simulink model "simulacaoESC2DOF_SIAC"  (R2015a)
settings: Solver=ode4  StartTime=0.0  StopTime=120  FixedStep=0.001  RelTol=1e-3
values from neighbouring files (symbols this model uses):
  ampSenoide = 20    [simuOrientacaoESC.m]
  ampSenoide2 = 20    [simuOrientacaoESC.m]
  freqSenoide = 4*2*pi    (= 25.1327412287)    [simuOrientacaoESC.m]
  K = 1    [simuOrientacaoESC.m]
  Kp = 10    [simuOrientacaoESC.m]
undefined symbols (not defined in the file or in its folder): xL0
libraries: simulink_extras x5
settings Model: Creator=Jean  LastModifiedBy=Jean

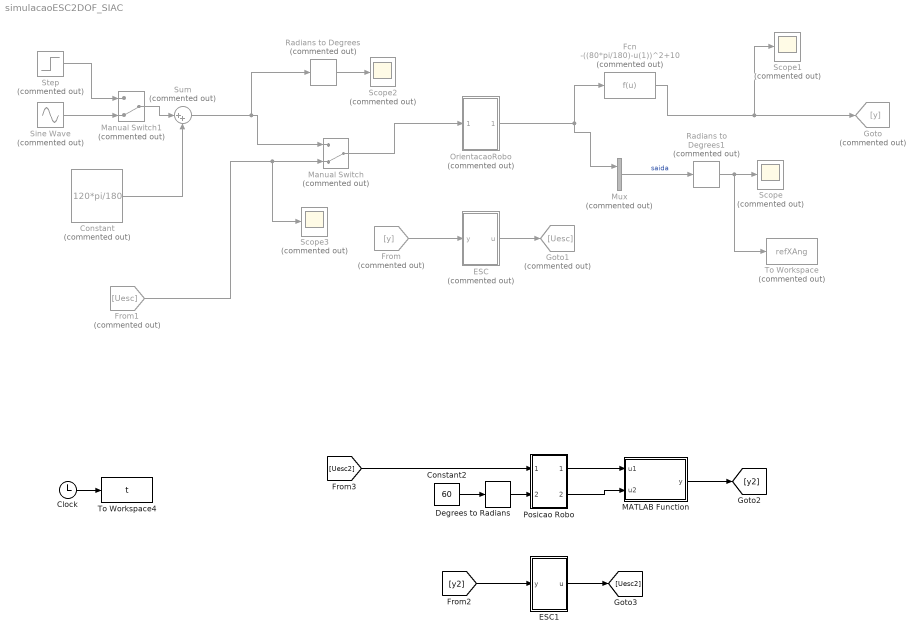
== system simulacaoESC2DOF_SIAC ==
  Clock : Clock
  Constant : Constant  Commented=on  Value=120*pi/180
  Constant2 : Constant  Value=60
  Degrees to Radians : simulink_extras/Transformations/Degrees to Radians
  ESC : Subsystem  Commented=on
  ESC1 : Subsystem
  Fcn : Fcn  Commented=on  Expr=-((80*pi/180)-u(1))^2+10
  From : From  Commented=on  GotoTag=y
  From1 : From  Commented=on  GotoTag=Uesc
  Goto : Goto  Commented=on  GotoTag=y
  Goto1 : Goto  Commented=on  GotoTag=Uesc
  MATLAB Function : MATLAB Function  TreatAsAtomicUnit=on
  Manual Switch : ManualSwitch  Commented=on  CurrentSetting=0
  Manual Switch1 : ManualSwitch  Commented=on  CurrentSetting=0
  Mux : Mux  Commented=on  Inputs=2
  "OrientacaoRobo " : Subsystem  Commented=on
  "Posicao Robo " : Subsystem
  Radians to Degrees : simulink_extras/Transformations/Radians to Degrees  Commented=on
  Radians to Degrees1 : simulink_extras/Transformations/Radians to Degrees  Commented=on
  Scope{,1..3} (4 alike) : Scope  Commented=on
      Scope settings: TimeRange=10  YMin=297  YMax=319
      Scope1 settings: TimeRange=10  YMin=5.5  YMax=10  SaveName=ScopeData2
      Scope2 settings: TimeRange=10  YMin=-60  YMax=60  SaveName=ScopeData3
      Scope3 settings: TimeRange=10  YMin=-60  YMax=60  SaveName=ScopeData4
  Sine Wave : Sin  Commented=on  Amplitude=60*pi/180  Frequency=180*pi/180  SampleTime=0
  Step : Step  Commented=on  SampleTime=0
  Sum : Sum  Commented=on  Inputs=|++
  To Workspace : ToWorkspace  Commented=on  VariableName=refXAng  SaveFormat=Structure With Time  SampleTime=-1
  To Workspace4 : ToWorkspace  VariableName=t  SampleTime=-1
  wires:
  Manual Switch/1 -> "OrientacaoRobo "/1(In1)
  Mux/1 -> Radians to Degrees1/1  "saida"
  From/1 -> ESC/1(y)
  ESC/1(u) -> Goto1/1
  From1/1 -> Scope3/1, Manual Switch/2
  Radians to Degrees/1 -> Scope2/1
  Sum/1 -> Radians to Degrees/1, Manual Switch/1
  Constant/1 -> Sum/2
  Radians to Degrees1/1 -> To Workspace/1, Scope/1
  "OrientacaoRobo "/1(Out1) -> Mux/1, Fcn/1
  Fcn/1 -> Scope1/1, Goto/1
  Step/1 -> Manual Switch1/1
  Sine Wave/1 -> Manual Switch1/2
  Manual Switch1/1 -> Sum/1
  [y2] -> ESC1/1(y)
  ESC1/1(u) -> [Uesc2]
  "Posicao Robo "/1(Out1) -> MATLAB Function/1(u1)
  MATLAB Function/1(y) -> [y2]
  [Uesc2] -> "Posicao Robo "/1(In1)
  Constant2/1 -> Degrees to Radians/1
  Degrees to Radians/1 -> "Posicao Robo "/2(In2)
  "Posicao Robo "/2(Out2) -> MATLAB Function/2(u2)
  Clock/1 -> To Workspace4/1

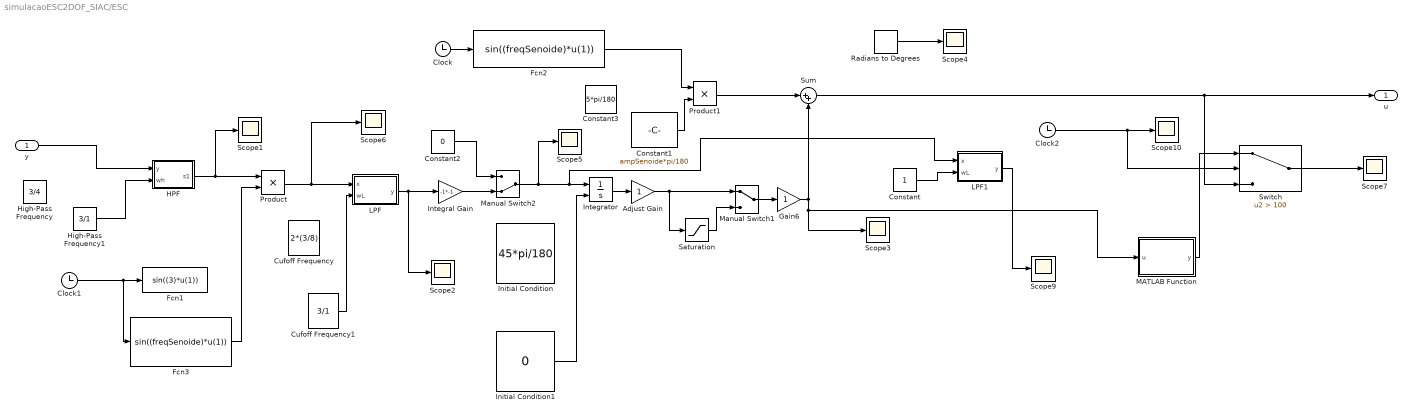
== system simulacaoESC2DOF_SIAC/ESC ==
  y : Inport
  Adjust Gain : Gain
  Clock : Clock
  Clock1 : Clock
  Clock2 : Clock
  Constant : Constant
  Constant1 : Constant  Value=ampSenoide*pi/180  SampleTime=Inf
  Constant2 : Constant  Value=0
  Constant3 : Constant  Value=5*pi/180  SampleTime=Inf
  Cufoff Frequency : Constant  Value=2*(3/8)  SampleTime=Inf
  Cufoff Frequency1 : Constant  Value=3/1  SampleTime=Inf
  Fcn1 : Fcn  Expr=sin((3)*u(1))
  Fcn2 : Fcn  Expr=sin((freqSenoide)*u(1))
  Fcn3 : Fcn  Expr=sin((freqSenoide)*u(1))
  Gain6 : Gain
  HPF : Subsystem
  High-Pass Frequency : Constant  Value=3/4  SampleTime=Inf
  High-Pass Frequency1 : Constant  Value=3/1  SampleTime=Inf
  Initial Condition : Constant  Value=45*pi/180  SampleTime=Inf
  Initial Condition1 : Constant  Value=0  SampleTime=Inf
  Integral Gain : Gain  Gain=-1*-1
  Integrator : Integrator  InitialConditionSource=external
  LPF : Subsystem
  LPF1 : Subsystem
  MATLAB Function : MATLAB Function  TreatAsAtomicUnit=on
  Manual Switch1 : ManualSwitch
  Manual Switch2 : ManualSwitch  CurrentSetting=0
  Product : Product
  Product1 : Product
  Radians to Degrees : simulink_extras/Transformations/Radians to Degrees
  Saturation : Saturate  UpperLimit=100  LowerLimit=-100
  Scope{1..7,9..10} (9 alike) : Scope
      Scope1 settings: YMin=-0.25  YMax=2.5  SaveName=ScopeData6
      Scope10 settings: TimeRange=10  YMin=-900  YMax=0  SaveName=ScopeData14
      Scope2 settings: YMin=-1  YMax=1  SaveName=ScopeData8
      Scope3 settings: TimeRange=10  YMin=-900  YMax=0  SaveName=ScopeData9
      Scope4 settings: TimeRange=10  YMin=0.375  YMax=0.65  SaveName=ScopeData10
      Scope5 settings: TimeRange=10  YMin=-1  YMax=1
      Scope6 settings: YMin=-0.2  YMax=0.25  SaveName=ScopeData7
      Scope7 settings: TimeRange=10  YMin=-900  YMax=0  SaveName=ScopeData11
      Scope9 settings: TimeRange=10  YMin=0.375  YMax=0.65  SaveName=ScopeData13
  Sum : Sum  Inputs=|++
  Switch : Switch  Criteria=u2 > Threshold  Threshold=100
  u : Outport
  wires:
  Product1/1 -> Sum/1
  Constant2/1 -> Manual Switch2/1
  Fcn2/1 -> Product1/1
  Integrator/1 -> Adjust Gain/1
  y/1 -> HPF/1(y)
  Gain6/1 -> MATLAB Function/1(u), Scope3/1, Sum/2
  Clock/1 -> Fcn2/1
  Clock1/1 -> Fcn3/1, Fcn1/1
  HPF/1(s1) -> Product/1, Scope1/1
  Adjust Gain/1 -> Saturation/1, Manual Switch1/1
  LPF/1(y) -> Integral Gain/1, Scope2/1
  Integral Gain/1 -> Manual Switch2/2
  Manual Switch1/1 -> Gain6/1
  Manual Switch2/1 -> Scope5/1, LPF1/1(x), Integrator/1
  Saturation/1 -> Manual Switch1/2
  Product/1 -> Scope6/1, LPF/1(x)
  High-Pass Frequency1/1 -> HPF/2(wh)
  Fcn3/1 -> Product/2
  Cufoff Frequency1/1 -> LPF/2(wL)
  Initial Condition1/1 -> Integrator/2
  Constant1/1 -> Product1/2
  Radians to Degrees/1 -> Scope4/1
  Constant/1 -> LPF1/2(wL)
  LPF1/1(y) -> Scope9/1
  Sum/1 -> u/1, Switch/3
  Switch/1 -> Scope7/1
  Clock2/1 -> Switch/2, Scope10/1
  MATLAB Function/1(y) -> Switch/1

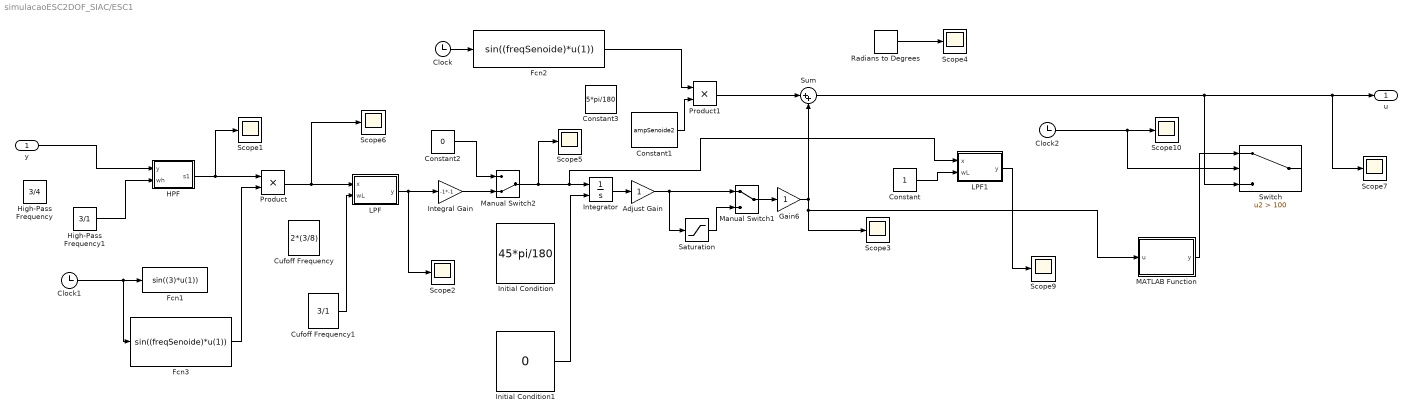
== system simulacaoESC2DOF_SIAC/ESC1 ==
  y : Inport
  Adjust Gain : Gain
  Clock : Clock
  Clock1 : Clock
  Clock2 : Clock
  Constant : Constant
  Constant1 : Constant  Value=ampSenoide2  SampleTime=Inf
  Constant2 : Constant  Value=0
  Constant3 : Constant  Value=5*pi/180  SampleTime=Inf
  Cufoff Frequency : Constant  Value=2*(3/8)  SampleTime=Inf
  Cufoff Frequency1 : Constant  Value=3/1  SampleTime=Inf
  Fcn1 : Fcn  Expr=sin((3)*u(1))
  Fcn2 : Fcn  Expr=sin((freqSenoide)*u(1))
  Fcn3 : Fcn  Expr=sin((freqSenoide)*u(1))
  Gain6 : Gain
  HPF : Subsystem
  High-Pass Frequency : Constant  Value=3/4  SampleTime=Inf
  High-Pass Frequency1 : Constant  Value=3/1  SampleTime=Inf
  Initial Condition : Constant  Value=45*pi/180  SampleTime=Inf
  Initial Condition1 : Constant  Value=0  SampleTime=Inf
  Integral Gain : Gain  Gain=-1*-1
  Integrator : Integrator  InitialConditionSource=external
  LPF : Subsystem
  LPF1 : Subsystem
  MATLAB Function : MATLAB Function  TreatAsAtomicUnit=on
  Manual Switch1 : ManualSwitch
  Manual Switch2 : ManualSwitch  CurrentSetting=0
  Product : Product
  Product1 : Product
  Radians to Degrees : simulink_extras/Transformations/Radians to Degrees
  Saturation : Saturate  UpperLimit=100  LowerLimit=-100
  Scope{1..7,9..10} (9 alike) : Scope
      Scope1 settings: YMin=-0.25  YMax=2.5  SaveName=ScopeData6
      Scope10 settings: TimeRange=10  YMin=-900  YMax=0  SaveName=ScopeData14
      Scope2 settings: YMin=-1  YMax=1  SaveName=ScopeData8
      Scope3 settings: TimeRange=10  YMin=-900  YMax=0  SaveName=ScopeData9
      Scope4 settings: TimeRange=10  YMin=0.375  YMax=0.65  SaveName=ScopeData10
      Scope5 settings: TimeRange=10  YMin=-1  YMax=1
      Scope6 settings: YMin=-0.2  YMax=0.25  SaveName=ScopeData7
      Scope7 settings: TimeRange=10  YMin=-900  YMax=0  SaveName=ScopeData11
      Scope9 settings: TimeRange=10  YMin=0.375  YMax=0.65  SaveName=ScopeData13
  Sum : Sum  Inputs=|++
  Switch : Switch  Criteria=u2 > Threshold  Threshold=100
  u : Outport
  wires:
  Product1/1 -> Sum/1
  Constant2/1 -> Manual Switch2/1
  Fcn2/1 -> Product1/1
  Integrator/1 -> Adjust Gain/1
  y/1 -> HPF/1(y)
  Gain6/1 -> MATLAB Function/1(u), Scope3/1, Sum/2
  Clock/1 -> Fcn2/1
  Clock1/1 -> Fcn3/1, Fcn1/1
  HPF/1(s1) -> Product/1, Scope1/1
  Adjust Gain/1 -> Saturation/1, Manual Switch1/1
  LPF/1(y) -> Integral Gain/1, Scope2/1
  Integral Gain/1 -> Manual Switch2/2
  Manual Switch1/1 -> Gain6/1
  Manual Switch2/1 -> Scope5/1, LPF1/1(x), Integrator/1
  Saturation/1 -> Manual Switch1/2
  Product/1 -> Scope6/1, LPF/1(x)
  High-Pass Frequency1/1 -> HPF/2(wh)
  Fcn3/1 -> Product/2
  Cufoff Frequency1/1 -> LPF/2(wL)
  Constant1/1 -> Product1/2
  Radians to Degrees/1 -> Scope4/1
  Constant/1 -> LPF1/2(wL)
  LPF1/1(y) -> Scope9/1
  Sum/1 -> u/1, Scope7/1, Switch/3
  Clock2/1 -> Switch/2, Scope10/1
  MATLAB Function/1(y) -> Switch/1
  Initial Condition1/1 -> Integrator/2

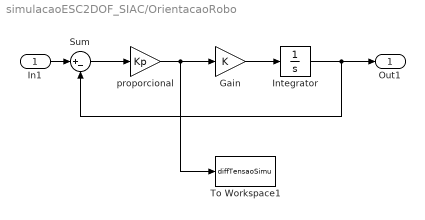
== system simulacaoESC2DOF_SIAC/OrientacaoRobo  ==
  In1 : Inport
  Gain : Gain  Gain=K
  Integrator : Integrator
  Sum : Sum  Inputs=|+-
  To Workspace1 : ToWorkspace  VariableName=diffTensaoSimu  SaveFormat=Structure With Time  SampleTime=-1
  "proporcional " : Gain  Gain=Kp
  Out1 : Outport
  wires:
  Gain/1 -> Integrator/1
  Integrator/1 -> Out1/1, Sum/2
  In1/1 -> Sum/1
  "proporcional "/1 -> To Workspace1/1, Gain/1
  Sum/1 -> "proporcional "/1

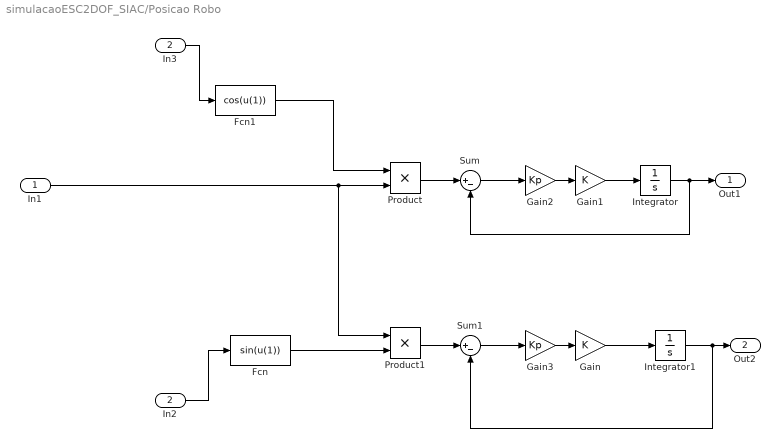
== system simulacaoESC2DOF_SIAC/Posicao Robo  ==
  In1 : Inport
  In2 : Inport  Port=2
  Fcn : Fcn  Expr=sin(u(1))
  Fcn1 : Fcn  Expr=cos(u(1))
  Gain : Gain  Gain=K
  Gain1 : Gain  Gain=K
  Gain2 : Gain  Gain=Kp
  Gain3 : Gain  Gain=Kp
  In3 : InportShadow  Port=2
  Integrator : Integrator
  Integrator1 : Integrator
  Product : Product
  Product1 : Product
  Sum : Sum  Inputs=|+-
  Sum1 : Sum  Inputs=|+-
  Out1 : Outport
  Out2 : Outport  Port=2
  wires:
  Integrator/1 -> Sum/2, Out1/1
  Integrator1/1 -> Sum1/2, Out2/1
  Fcn/1 -> Product1/2
  In2/1 -> Fcn/1
  In3/1 -> Fcn1/1
  Fcn1/1 -> Product/1
  Gain/1 -> Integrator1/1
  Gain1/1 -> Integrator/1
  In1/1 -> Product1/1, Product/2
  Product/1 -> Sum/1
  Sum/1 -> Gain2/1
  Product1/1 -> Sum1/1
  Sum1/1 -> Gain3/1
  Gain2/1 -> Gain1/1
  Gain3/1 -> Gain/1

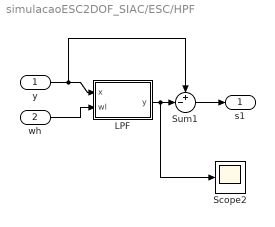
== system simulacaoESC2DOF_SIAC/ESC/HPF ==
  y : Inport
  wh : Inport  Port=2
  LPF : Subsystem
  Scope2 : Scope
      settings: YMin=0.6  YMax=1.125  SaveName=ScopeData5
  Sum1 : Sum  Inputs=+-|
  s1 : Outport
  wires:
  LPF/1(y) -> Sum1/2, Scope2/1
  wh/1 -> LPF/2(wl)
  Sum1/1 -> s1/1
  y/1 -> Sum1/1, LPF/1(x)

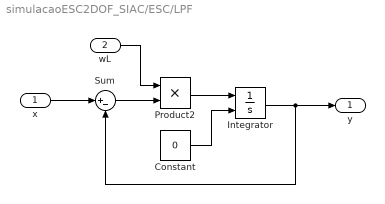
== system simulacaoESC2DOF_SIAC/ESC/LPF ==
  x : Inport
  wL : Inport  Port=2
  Constant : Constant  Value=0
  Integrator : Integrator  InitialConditionSource=external  InitialCondition=xL0
  Product2 : Product
  Sum : Sum  Inputs=|+-
  y : Outport
  wires:
  Constant/1 -> Integrator/2
  x/1 -> Sum/1
  Sum/1 -> Product2/2
  Product2/1 -> Integrator/1
  Integrator/1 -> y/1, Sum/2
  wL/1 -> Product2/1

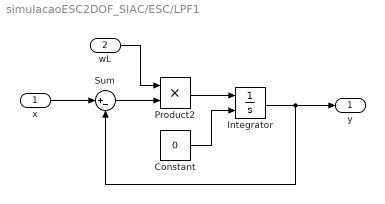
== system simulacaoESC2DOF_SIAC/ESC/LPF1 ==
  x : Inport
  wL : Inport  Port=2
  Constant : Constant  Value=0
  Integrator : Integrator  InitialConditionSource=external  InitialCondition=xL0
  Product2 : Product
  Sum : Sum  Inputs=|+-
  y : Outport
  wires:
  Constant/1 -> Integrator/2
  x/1 -> Sum/1
  Sum/1 -> Product2/2
  Product2/1 -> Integrator/1
  Integrator/1 -> y/1, Sum/2
  wL/1 -> Product2/1

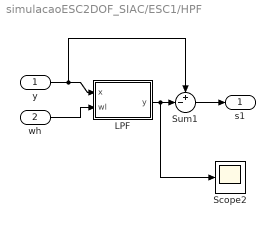
== system simulacaoESC2DOF_SIAC/ESC1/HPF ==
  y : Inport
  wh : Inport  Port=2
  LPF : Subsystem
  Scope2 : Scope
      settings: YMin=0.6  YMax=1.125  SaveName=ScopeData5
  Sum1 : Sum  Inputs=+-|
  s1 : Outport
  wires:
  LPF/1(y) -> Sum1/2, Scope2/1
  wh/1 -> LPF/2(wl)
  Sum1/1 -> s1/1
  y/1 -> Sum1/1, LPF/1(x)

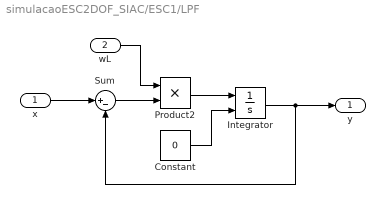
== system simulacaoESC2DOF_SIAC/ESC1/LPF ==
  x : Inport
  wL : Inport  Port=2
  Constant : Constant  Value=0
  Integrator : Integrator  InitialConditionSource=external  InitialCondition=xL0
  Product2 : Product
  Sum : Sum  Inputs=|+-
  y : Outport
  wires:
  Constant/1 -> Integrator/2
  x/1 -> Sum/1
  Sum/1 -> Product2/2
  Product2/1 -> Integrator/1
  Integrator/1 -> y/1, Sum/2
  wL/1 -> Product2/1

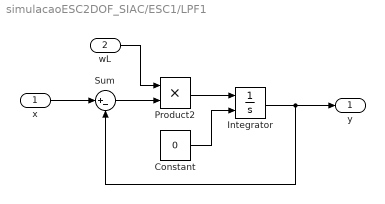
== system simulacaoESC2DOF_SIAC/ESC1/LPF1 ==
  x : Inport
  wL : Inport  Port=2
  Constant : Constant  Value=0
  Integrator : Integrator  InitialConditionSource=external  InitialCondition=xL0
  Product2 : Product
  Sum : Sum  Inputs=|+-
  y : Outport
  wires:
  Constant/1 -> Integrator/2
  x/1 -> Sum/1
  Sum/1 -> Product2/2
  Product2/1 -> Integrator/1
  Integrator/1 -> y/1, Sum/2
  wL/1 -> Product2/1

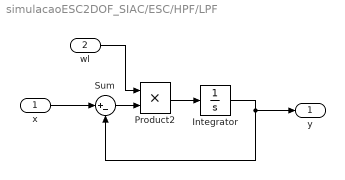
== system simulacaoESC2DOF_SIAC/ESC/HPF/LPF ==
  x : Inport
  wl : Inport  Port=2
  Integrator : Integrator
  Product2 : Product
  Sum : Sum  Inputs=|+-
  y : Outport
  wires:
  wl/1 -> Product2/1
  Integrator/1 -> y/1, Sum/2
  Product2/1 -> Integrator/1
  Sum/1 -> Product2/2
  x/1 -> Sum/1

== system simulacaoESC2DOF_SIAC/ESC1/HPF/LPF ==
  x : Inport
  wl : Inport  Port=2
  Integrator : Integrator
  Product2 : Product
  Sum : Sum  Inputs=|+-
  y : Outport
  wires:
  wl/1 -> Product2/1
  Integrator/1 -> y/1, Sum/2
  Product2/1 -> Integrator/1
  Sum/1 -> Product2/2
  x/1 -> Sum/1

== matlab function simulacaoESC2DOF_SIAC/ESC1/MATLAB Function ==
  data: u input; y output
function y = fcn(u)
menorValor = 5;
if(abs(u)<menorValor)
    menorValor = u;
end

y = menorValor;

== matlab function simulacaoESC2DOF_SIAC/ESC/MATLAB Function ==
  data: u input; y output
function y = fcn(u)
menorValor = 5;
if(abs(u)<menorValor)
    menorValor = u;
end

y = menorValor;

== matlab function simulacaoESC2DOF_SIAC/MATLAB Function ==
  data: u1 input; y output; u2 input
function y = fcn(u1,u2)
%#codegen
%vetorDistancia = sqrt(u1^2+u2^2);
%exp = -((vetorDistancia-80)^2)/10+10;
exp = (-((u1-50)^2+(u2-86.60)^2))/10+10;

y = exp;
